simulink model "rrc_dob_voltage_compensation_wrapper"  (R2026a)
settings: Solver=FixedStepDiscrete  FixedStep=5e-5
settings Model: Creator=ASUS  LastModifiedBy=ASUS
settings HardwareCC: ProdLargestAtomicInteger=Long  ProdLargestAtomicFloat=Double  ProdHWDeviceType=ARM Compatible->ARM Cortex
settings RTWCC: SystemTargetFile=ert.tlc  GenCodeOnly=on  Description=Embedded Coder
settings ERTTargetCC: GenerateSampleERTMain=on  SupportNonFinite=off

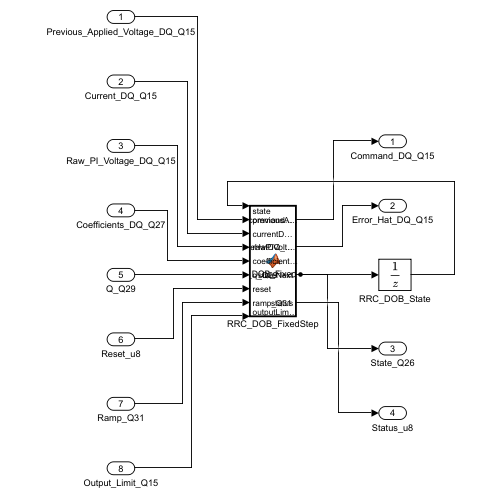
[thumbnail: Simulink's stored preview of the top-level diagram]
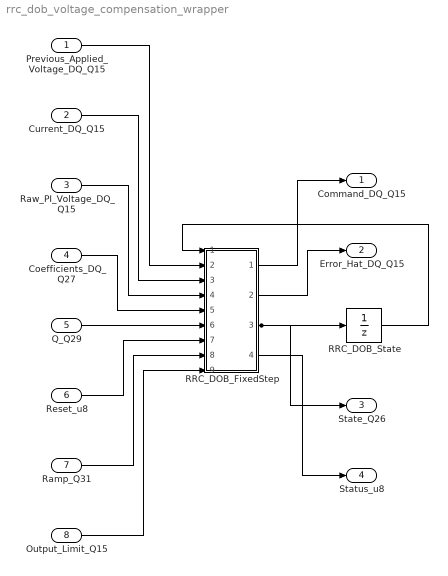
== system rrc_dob_voltage_compensation_wrapper ==
  Previous_Applied_Voltage_DQ_Q15 : Inport  OutDataTypeStr=int16  PortDimensions=2
  Current_DQ_Q15 : Inport  Port=2  OutDataTypeStr=int16  PortDimensions=2
  Raw_PI_Voltage_DQ_Q15 : Inport  Port=3  OutDataTypeStr=int16  PortDimensions=2
  Coefficients_DQ_Q27 : Inport  Port=4  OutDataTypeStr=int32  PortDimensions=[19 2]
  Q_Q29 : Inport  Port=5  OutDataTypeStr=int32  PortDimensions=1
  Reset_u8 : Inport  Port=6  OutDataTypeStr=uint8  PortDimensions=1
  Ramp_Q31 : Inport  Port=7  OutDataTypeStr=uint32  PortDimensions=1
  Output_Limit_Q15 : Inport  Port=8  OutDataTypeStr=int16  PortDimensions=1
  RRC_DOB_FixedStep : MATLAB Function  TreatAsAtomicUnit=on
  RRC_DOB_State : UnitDelay  InitialCondition=zeros(8,1,'int32')  SampleTime=5e-5
  Command_DQ_Q15 : Outport
  Error_Hat_DQ_Q15 : Outport  Port=2
  State_Q26 : Outport  Port=3
  Status_u8 : Outport  Port=4
  wires:
  RRC_DOB_State/1 -> RRC_DOB_FixedStep/1(state)
  Previous_Applied_Voltage_DQ_Q15/1 -> RRC_DOB_FixedStep/2(previousAppliedVoltageDQ_Q15)
  Current_DQ_Q15/1 -> RRC_DOB_FixedStep/3(currentDQ_Q15)
  Raw_PI_Voltage_DQ_Q15/1 -> RRC_DOB_FixedStep/4(rawPiVoltageDQ_Q15)
  Coefficients_DQ_Q27/1 -> RRC_DOB_FixedStep/5(coefficientsDQ_Q27)
  Q_Q29/1 -> RRC_DOB_FixedStep/6(q_Q29)
  Reset_u8/1 -> RRC_DOB_FixedStep/7(reset)
  Ramp_Q31/1 -> RRC_DOB_FixedStep/8(ramp_Q31)
  Output_Limit_Q15/1 -> RRC_DOB_FixedStep/9(outputLimit_Q15)
  RRC_DOB_FixedStep/1(commandDQ_Q15) -> Command_DQ_Q15/1
  RRC_DOB_FixedStep/2(eHatDQ_Q15) -> Error_Hat_DQ_Q15/1
  RRC_DOB_FixedStep/3(stateNext) -> State_Q26/1, RRC_DOB_State/1
  RRC_DOB_FixedStep/4(status) -> Status_u8/1

== matlab function rrc_dob_voltage_compensation_wrapper/RRC_DOB_FixedStep ==
  data: state input int32 size=[8 1]; commandDQ_Q15 output int16 size=[2 1]; previousAppliedVoltageDQ_Q15 input int16 size=[2 1]; currentDQ_Q15 input int16 size=[2 1]; rawPiVoltageDQ_Q15 input int16 size=[2 1]; coefficientsDQ_Q27 input int32 size=[19 2]; q_Q29 input int32 size=1; reset input uint8 size=1; ramp_Q31 input uint32 size=1; outputLimit_Q15 input int16 size=1; eHatDQ_Q15 output int16 size=[2 1]; stateNext output int32 size=[8 1]; status output uint8 size=1
function [commandDQ_Q15, eHatDQ_Q15, stateNext, status] = RRC_DOB_FixedStep(state, previousAppliedVoltageDQ_Q15, currentDQ_Q15, rawPiVoltageDQ_Q15, coefficientsDQ_Q27, q_Q29, reset, ramp_Q31, outputLimit_Q15)
%#codegen
[commandDQ_Q15, eHatDQ_Q15, stateNext, status] = rrcDobFixedPointStep(state, previousAppliedVoltageDQ_Q15, currentDQ_Q15, rawPiVoltageDQ_Q15, coefficientsDQ_Q27, q_Q29, reset, ramp_Q31, outputLimit_Q15);
end
